simulink model "VSC_Grid_MyModel"  (R2017b)
settings: Solver=VariableStepAuto  StartTime=0.0  StopTime=5  MaxStep=1e-4  RelTol=1e-3  AbsTol=1e-3
PreLoadFcn:
  | VSC_Grid_Data_MyModel
values from neighbouring files (symbols this model uses):
  alpha_PQ = alpha_cc/10    (= 314.159265359)    [VSC_Grid_Data_MyModel.m]
  C_dc = 5000e-06    (= 0.005)    [VSC_Grid_Data_MyModel.m]
  D_low = 0.0001    [VSC_Grid_Data_MyModel.m]
  D_up = 0.9999    [VSC_Grid_Data_MyModel.m]
  fn = 50    [VSC_Grid_Data_MyModel.m]
  fnmax = 51    [VSC_Grid_Data_MyModel.m]
  fnmin = 49    [VSC_Grid_Data_MyModel.m]
  Kp_cc = alpha_cc*Lf    (= 6.28318530718)    [VSC_Grid_Data_MyModel.m]
  Kp_PLL = alpha_PLL*2    (= 62.8318530718)    [VSC_Grid_Data_MyModel.m]
  Lf = 2e-3    (= 0.002)    [VSC_Grid_Data_MyModel.m]
  R_dc = 1e-5    (= 1e-05)    [VSC_Grid_Data_MyModel.m]
  Rf = 6e-3    (= 0.006)    [VSC_Grid_Data_MyModel.m]
  samp_delay = 1.5*Ts    (= 0.0003)    [VSC_Grid_Data_MyModel.m]
  Ts = 2e-4    (= 0.0002)    [VSC_Grid_Data_MyModel.m]
  V_dc = 680    [VSC_Grid_Data_MyModel.m]
  VLL_rms = 230*sqrt(3)    [VSC_Grid_Data_MyModel.m]
undefined symbols (not defined in the file or in its folder): DiscIntNeverNeededParam, sigbuilder_block
libraries: powerlib x9, powerlib_meascontrol x4
settings Model: Creator=saioa  LastModifiedBy=saioa
settings DataIOCC: SaveFormat=Array  SaveOutput=off  SaveTime=off
settings OptimizationCC: LifeSpan=inf
settings DebuggingCC: UnconnectedInputMsg=none  UnconnectedOutputMsg=none  UnconnectedLineMsg=none

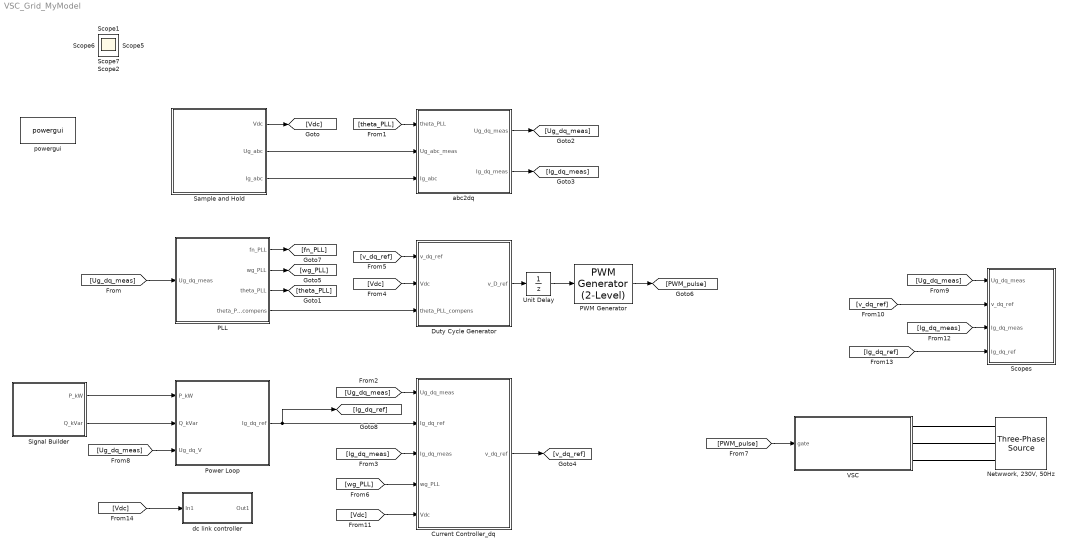
== system VSC_Grid_MyModel ==
  Current Controller_dq : Subsystem
  Duty Cycle Generator : Subsystem
  "Netwwork, 230V, 50Hz" : powerlib/Electrical Sources/Three-Phase Source  InternalConnection=Yg  VoltagePhases=off  Voltage=VLL_rms  PhaseAngle=0  Voltage_phases=[25e3 25e3 25e3]/sqrt(3)  PhaseAngles_phases=[0 -120 +120]  Frequency=fn  NonIdealSource=off  SpecifyImpedance=on  Resistance=0.8929  Inductance=16.58e-3  ShortCircuitLevel=40e6  BaseVoltage=600  XRratio=7  BusType=swing  Pref=0  Qref=0  Prefabc=[10e3, 10e3, 10e3]  Qrefabc=[0, 0, 0]  Qmin=-inf  Qmax=inf
  PLL : Subsystem
  PWM Generator : powerlib_meascontrol/Pulse & Signal Generators/PWM Generator (2-Level)  ModulatorType=Three-phase bridge (6 pulses)  ModulatorMode=Unsynchronized  Fc=fs  Pc=0  nF=27  MinMax="[ -1  1 ]"  SamplingTechnique=Symmetrical regular (single edge)  ModulatingSignals=off  m=0.8  Freq=60  Phase=0  Ts=0  ShowCarrierOutport=off
      settings: SourceProductName=Simscape Power Systems
  Power Loop : Subsystem
  Sample and Hold : Subsystem
  Scopes : Subsystem
  Signal Builder : Subsystem  Tag=STV Subsys  LoadFcn=sigbuilder_block('load');  StartFcn=sigbuilder_block('start');  StopFcn=sigbuilder_block('stop');  ClipboardFcn=sigbuilder_block('clipboard');  mask(Sigbuilder block){tuvar=[0:10]}
      mask help: Simulink:masks:SigbuilderBlock_MD
      mask init:
      | if ~strcmp(get_param(bdroot(gcbh),'SimulationStatus'),'stopped') tuvar = sigbuilder_block('maskInit'); end
      settings: CopyFcn=sigbuilder_block('copy');  DeleteFcn=sigbuilder_block('delete');  ModelCloseFcn=sigbuilder_block('modelClose');  PreSaveFcn=sigbuilder_block('preSave');  PauseFcn=sigbuilder_block('pause');  ContinueFcn=sigbuilder_block('continue');  NameChangeFcn=sigbuilder_block('namechange');  OpenFcn=sigbuilder_block('open',[6 33 1428 678 ]);  CloseFcn=sigbuilder_block('close');
      mask Display: plot(0, 0, 100, 100,[2, 2, 32, 32, 2], [68, 8, 8, 68, 68],[32, 2], [38, 38], [32, 19, 2],[53, 60, 44], [32, 17, 17, 2],[16, 16, 31, 31]);txt = getActiveGroup(gcbh);text(2, 100, txt,'verticalAlignment', 'top');
  Unit Delay : UnitDelay  SampleTime=-1
  VSC : Subsystem
  "abc2dq " : Subsystem
  dc link controller : Subsystem
  powergui : powerlib/powergui  Priority=1  SimulationMode=Continuous  SampleTime=50e-6  frequency=60  Iterations=50  frequencyindice=50  Pbase=100e6  ErrMax=1e-4  UnitsV=kV  UnitsW=MW  buscounter=0  FunctionMessages=off  echomessages=off  EnableUseOfTLC=off  CurrentSourceSwitches=off  DisableSnubberDevices=off  DisableRonSwitches=off  DisableVfSwitches=off  DisplayEquations=off  SolverType=Tustin/Backward Euler (TBE)  Interpol=off  ExternalGateDelay=off  methode=off  Ts=100  x0status=blocks  SPID=on  SwTol=0  HookPort=off  RestoreLinks=warning  ResistiveCurrentMeasurement=off  Frange=[0:2:500]  Ylog=off  Xlog=on  ShowGrid=off  save=off  variable=ZData  structure=0  ZoomFFT=off  StartTime=0.0  cycles=1  DisplayStyle=1  fundamental=60  FreqAxis=off  MaxFrequency=1000  frequencyindicesteady=1  RmsSteady=1  display=off
  Scope{,1..2,5..7} (6 alike) : Scope
  wires:
  "abc2dq "/2(Ig_dq_meas) -> [Ig_dq_meas]
  Sample and Hold/1(Vdc) -> [Vdc]
  Sample and Hold/3(Ig_abc) -> "abc2dq "/3(Ig_abc)
  [v_dq_ref] -> Duty Cycle Generator/1(v_dq_ref)
  PLL/4(theta_PLL_compens) -> Duty Cycle Generator/3(theta_PLL_compens)
  Current Controller_dq/1(v_dq_ref) -> [v_dq_ref]
  [Vdc] -> Duty Cycle Generator/2(Vdc)
  [Ug_dq_meas] -> Current Controller_dq/1(Ug_dq_meas)
  [theta_PLL] -> "abc2dq "/1(theta_PLL)
  "abc2dq "/1(Ug_dq_meas) -> [Ug_dq_meas]
  PLL/2(wg_PLL) -> [wg_PLL]
  [wg_PLL] -> Current Controller_dq/4(wg_PLL)
  PLL/1(fn_PLL) -> [fn_PLL]
  Sample and Hold/2(Ug_abc) -> "abc2dq "/2(Ug_abc_meas)
  PLL/3(theta_PLL) -> [theta_PLL]
  [Ug_dq_meas] -> PLL/1(Ug_dq_meas)
  [PWM_pulse] -> VSC/1(gate)
  Signal Builder/1(P_kW) -> Power Loop/1(P_kW)
  Signal Builder/2(Q_kVar) -> Power Loop/2(Q_kVar)
  [Ug_dq_meas] -> Power Loop/3(Ug_dq_V)
  Power Loop/1(Ig_dq_ref) -> Current Controller_dq/2(Ig_dq_ref), [Ig_dq_ref]
  [Ig_dq_meas] -> Current Controller_dq/3(Ig_dq_meas)
  [Vdc] -> Current Controller_dq/5(Vdc)
  PWM Generator/1 -> [PWM_pulse]
  Duty Cycle Generator/1(v_D_ref) -> Unit Delay/1
  Unit Delay/1 -> PWM Generator/1
  [Ug_dq_meas] -> Scopes/1(Ug_dq_meas)
  [v_dq_ref] -> Scopes/2(v_dq_ref)
  [Ig_dq_meas] -> Scopes/3(Ig_dq_meas)
  [Ig_dq_ref] -> Scopes/4(Ig_dq_ref)
  [Vdc] -> dc link controller/1(In1)
  connections:
  "Netwwork, 230V, 50Hz"/RConn1 -- VSC/RConn1
  "Netwwork, 230V, 50Hz"/RConn2 -- VSC/RConn2
  "Netwwork, 230V, 50Hz"/RConn3 -- VSC/RConn3

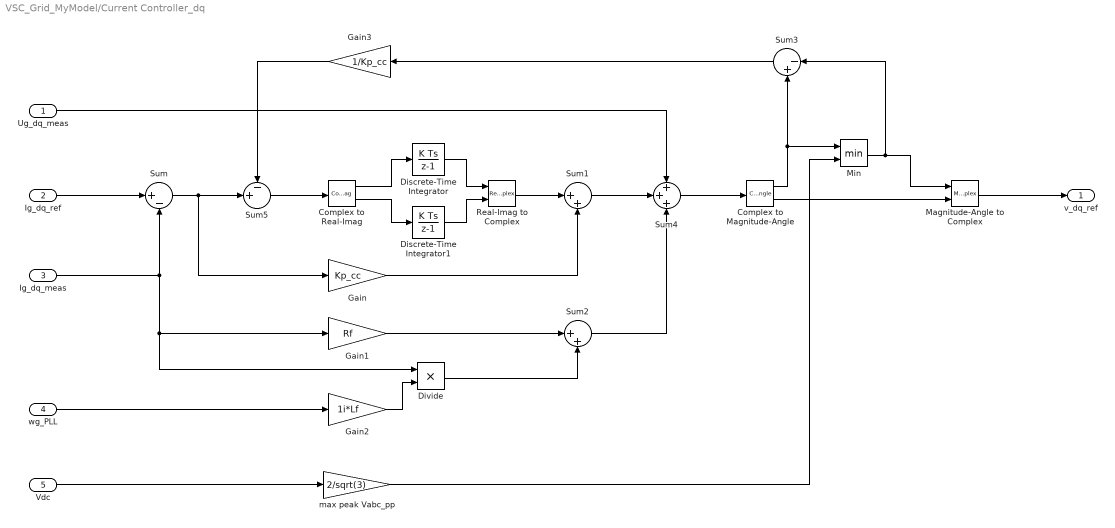
== system VSC_Grid_MyModel/Current Controller_dq ==
  Ug_dq_meas : Inport
  Ig_dq_ref : Inport  Port=2
  Ig_dq_meas : Inport  Port=3
  wg_PLL : Inport  Port=4
  Vdc : Inport  Port=5
  Complex to Magnitude-Angle : ComplexToMagnitudeAngle
  Complex to Real-Imag : ComplexToRealImag
  Discrete-Time Integrator : DiscreteIntegrator  gainval=Ki_cc  InitialConditionSetting=State (most efficient)  SampleTime=Ts  ICPrevOutput=DiscIntNeverNeededParam  ICPrevScaledInput=DiscIntNeverNeededParam
  Discrete-Time Integrator1 : DiscreteIntegrator  gainval=Ki_cc  InitialConditionSetting=State (most efficient)  SampleTime=Ts  ICPrevOutput=DiscIntNeverNeededParam  ICPrevScaledInput=DiscIntNeverNeededParam
  Divide : Product  Inputs=**
  Gain : Gain  Gain=Kp_cc
  Gain1 : Gain  Gain=Rf
  Gain2 : Gain  Gain=1i*Lf
  Gain3 : Gain  Gain=1/Kp_cc
  Magnitude-Angle to Complex : MagnitudeAngleToComplex
  Min : MinMax  Inputs=2
  Real-Imag to Complex : RealImagToComplex
  Sum : Sum  Inputs=|+-
  Sum1 : Sum  Inputs=|++
  Sum2 : Sum  Inputs=|++
  Sum3 : Sum  Inputs=|-+
  Sum4 : Sum  Inputs=+++  SaturateOnIntegerOverflow=on  InputSameDT=on  OutDataTypeStr=Inherit: Same as first input
  Sum5 : Sum  Inputs=-+|
  max peak Vabc_pp : Gain  Gain=2/sqrt(3)
  v_dq_ref : Outport
  wires:
  Ig_dq_meas/1 -> Gain1/1, Divide/1, Sum/2
  Ig_dq_ref/1 -> Sum/1
  Discrete-Time Integrator1/1 -> Real-Imag to Complex/2
  wg_PLL/1 -> Gain2/1
  Gain/1 -> Sum1/2
  Complex to Real-Imag/2 -> Discrete-Time Integrator1/1
  Discrete-Time Integrator/1 -> Real-Imag to Complex/1
  Real-Imag to Complex/1 -> Sum1/1
  Complex to Real-Imag/1 -> Discrete-Time Integrator/1
  Sum1/1 -> Sum4/2
  Sum2/1 -> Sum4/3
  Divide/1 -> Sum2/2
  Ug_dq_meas/1 -> Sum4/1
  Gain2/1 -> Divide/2
  Gain1/1 -> Sum2/1
  Vdc/1 -> max peak Vabc_pp/1
  Sum4/1 -> Complex to Magnitude-Angle/1
  Complex to Magnitude-Angle/1 -> Min/1, Sum3/2
  max peak Vabc_pp/1 -> Min/2
  Complex to Magnitude-Angle/2 -> Magnitude-Angle to Complex/2
  Min/1 -> Sum3/1, Magnitude-Angle to Complex/1
  Magnitude-Angle to Complex/1 -> v_dq_ref/1
  Sum5/1 -> Complex to Real-Imag/1
  Sum/1 -> Gain/1, Sum5/2
  Sum3/1 -> Gain3/1
  Gain3/1 -> Sum5/1

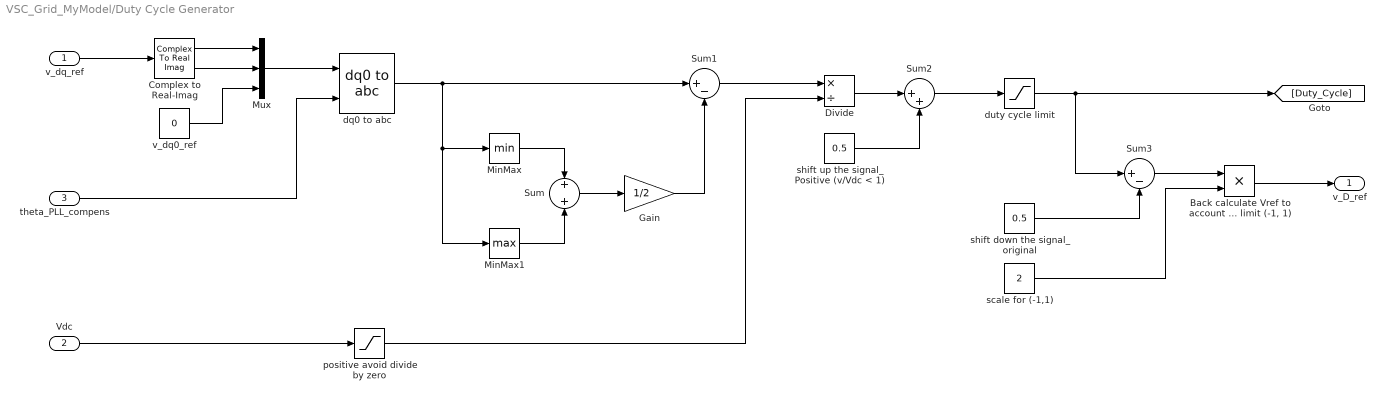
== system VSC_Grid_MyModel/Duty Cycle Generator ==
  v_dq_ref : Inport
  Vdc : Inport  Port=2
  theta_PLL_compens : Inport  Port=3
  "Back calculate Vref to account for duty cycle limit (-1, 1)" : Product  Inputs=**
  Complex to Real-Imag : ComplexToRealImag
  Divide : Product  Inputs=*/
  Gain : Gain  Gain=1/2
  MinMax : MinMax
  MinMax1 : MinMax  Function=max
  Mux : Mux  Inputs=3
  Sum : Sum  Inputs=+|+
  Sum1 : Sum  Inputs=|+-
  Sum2 : Sum  Inputs=|++
  Sum3 : Sum  Inputs=|+-
  dq0 to abc : powerlib_meascontrol/Transformations/dq0 to abc  Alignment=90 degrees behind phase A axis
  duty cycle limit : Saturate  UpperLimit=D_up  LowerLimit=D_low
  positive avoid divide by zero : Saturate  UpperLimit=inf  LowerLimit=1e-6
  scale for (-1,1) : Constant  Value=2
  shift down the signal_original : Constant  Value=0.5
  shift up the signal_Positive (v/Vdc < 1) : Constant  Value=0.5
  v_dq0_ref : Constant  Value=0
  v_D_ref : Outport
  wires:
  v_dq_ref/1 -> Complex to Real-Imag/1
  Complex to Real-Imag/1 -> Mux/1
  Complex to Real-Imag/2 -> Mux/2
  v_dq0_ref/1 -> Mux/3
  Mux/1 -> dq0 to abc/1
  theta_PLL_compens/1 -> dq0 to abc/2
  dq0 to abc/1 -> Sum1/1, MinMax1/1, MinMax/1
  Sum/1 -> Gain/1
  MinMax1/1 -> Sum/2
  MinMax/1 -> Sum/1
  Gain/1 -> Sum1/2
  Sum1/1 -> Divide/1
  Vdc/1 -> positive avoid divide by zero/1
  Divide/1 -> Sum2/1
  shift up the signal_Positive (v/Vdc < 1)/1 -> Sum2/2
  Sum2/1 -> duty cycle limit/1
  positive avoid divide by zero/1 -> Divide/2
  duty cycle limit/1 -> Sum3/1, [Duty_Cycle]
  shift down the signal_original/1 -> Sum3/2
  Sum3/1 -> "Back calculate Vref to account for duty cycle limit (-1, 1)"/1
  scale for (-1,1)/1 -> "Back calculate Vref to account for duty cycle limit (-1, 1)"/2
  "Back calculate Vref to account for duty cycle limit (-1, 1)"/1 -> v_D_ref/1

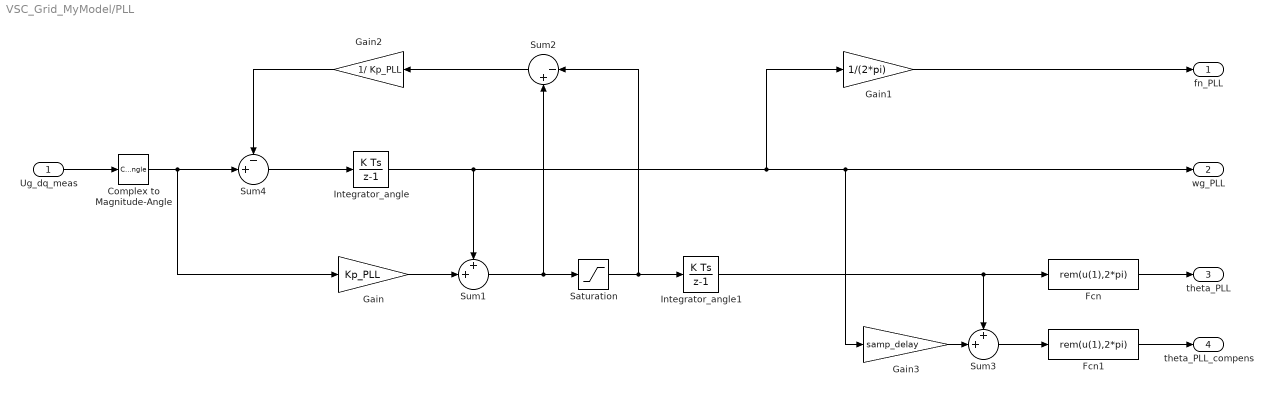
== system VSC_Grid_MyModel/PLL ==
  Ug_dq_meas : Inport
  Complex to Magnitude-Angle : ComplexToMagnitudeAngle  Output=Angle
  Fcn : Fcn  Expr=rem(u(1),2*pi)
  Fcn1 : Fcn  Expr=rem(u(1),2*pi)
  Gain : Gain  Gain=Kp_PLL
  Gain1 : Gain  Gain=1/(2*pi)
  Gain2 : Gain  Gain=1/ Kp_PLL
  Gain3 : Gain  Gain=samp_delay
  Integrator_angle : DiscreteIntegrator  gainval=Ki_PLL  InitialCondition=2*pi*fn  InitialConditionSetting=State (most efficient)  SampleTime=Ts  ICPrevOutput=DiscIntNeverNeededParam  ICPrevScaledInput=DiscIntNeverNeededParam
  Integrator_angle1 : DiscreteIntegrator  gainval=1  InitialConditionSetting=State (most efficient)  SampleTime=Ts  ICPrevOutput=DiscIntNeverNeededParam  ICPrevScaledInput=DiscIntNeverNeededParam
  Saturation : Saturate  UpperLimit=2*pi*fnmax  LowerLimit=2*pi*fnmin
  Sum1 : Sum  Inputs=++|
  Sum2 : Sum  Inputs=|-+
  Sum3 : Sum  Inputs=++|
  Sum4 : Sum  Inputs=-+|
  fn_PLL : Outport
  wg_PLL : Outport  Port=2
  theta_PLL : Outport  Port=3
  theta_PLL_compens : Outport  Port=4
  wires:
  Ug_dq_meas/1 -> Complex to Magnitude-Angle/1
  Integrator_angle/1 -> Gain1/1, wg_PLL/1, Gain3/1, Sum1/1
  Complex to Magnitude-Angle/1 -> Sum4/2, Gain/1
  Sum1/1 -> Sum2/2, Saturation/1
  Gain/1 -> Sum1/2
  Integrator_angle1/1 -> Sum3/1, Fcn/1
  Gain1/1 -> fn_PLL/1
  Fcn/1 -> theta_PLL/1
  Sum3/1 -> Fcn1/1
  Gain3/1 -> Sum3/2
  Fcn1/1 -> theta_PLL_compens/1
  Saturation/1 -> Sum2/1, Integrator_angle1/1
  Sum2/1 -> Gain2/1
  Sum4/1 -> Integrator_angle/1
  Gain2/1 -> Sum4/1

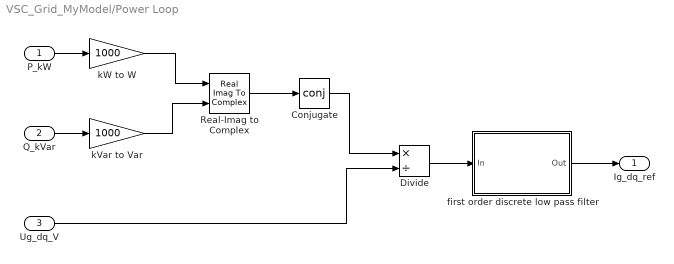
== system VSC_Grid_MyModel/Power Loop ==
  P_kW : Inport
  Q_kVar : Inport  Port=2
  Ug_dq_V : Inport  Port=3
  Conjugate : Math  Operator=conj  RndMeth=Zero  SaturateOnIntegerOverflow=on
  Divide : Product  Inputs=*/
  Real-Imag to Complex : RealImagToComplex
  first order discrete low pass filter : Subsystem  mask(First-order low pass filter (Discrete)){alpha_wfilter=alpha_PQ, Ts=Ts, Init=0}
      mask prompts: alpha_wfilter "Bandwidth (rad/s)"; Ts "Sampling time (>0, s)"; Init "Initial condition"
      mask help: Forward Euler method
  kVar to Var : Gain  Gain=1000
  kW to W : Gain  Gain=1000
  Ig_dq_ref : Outport
  wires:
  Divide/1 -> first order discrete low pass filter/1(In)
  Real-Imag to Complex/1 -> Conjugate/1
  Q_kVar/1 -> kVar to Var/1
  P_kW/1 -> kW to W/1
  Ug_dq_V/1 -> Divide/2
  Conjugate/1 -> Divide/1
  kW to W/1 -> Real-Imag to Complex/1
  kVar to Var/1 -> Real-Imag to Complex/2
  first order discrete low pass filter/1(Out) -> Ig_dq_ref/1

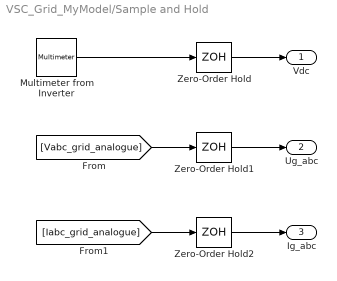
== system VSC_Grid_MyModel/Sample and Hold ==
  "Multimeter from Inverter " : powerlib/Measurements/Multimeter  PhasorSimulation=off  OutputType=Complex  sel=10  L=16  Gain=1  yselected="{'Udc: VSC/PWM  IGBT Inverter'};"  PSBOutputType=1  PSBequivalent=0  AxesSetting=[0,0.1,-100,100]  Display=0  SavedBlockNames=-11
  Zero-Order Hold : ZeroOrderHold  SampleTime=Ts
  Zero-Order Hold1 : ZeroOrderHold  SampleTime=Ts
  Zero-Order Hold2 : ZeroOrderHold  SampleTime=Ts
  Vdc : Outport
  Ug_abc : Outport  Port=2
  Ig_abc : Outport  Port=3
  wires:
  Zero-Order Hold/1 -> Vdc/1
  "Multimeter from Inverter "/1 -> Zero-Order Hold/1
  [Vabc_grid_analogue] -> Zero-Order Hold1/1
  [Iabc_grid_analogue] -> Zero-Order Hold2/1
  Zero-Order Hold1/1 -> Ug_abc/1
  Zero-Order Hold2/1 -> Ig_abc/1

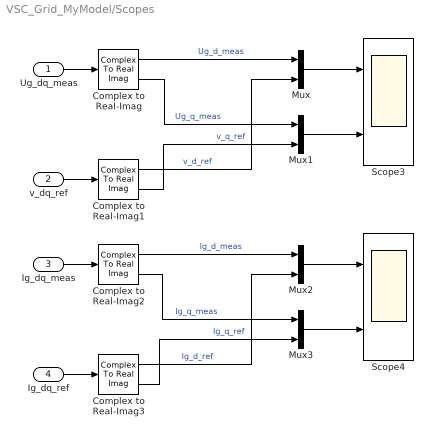
== system VSC_Grid_MyModel/Scopes ==
  Ug_dq_meas : Inport
  v_dq_ref : Inport  Port=2
  Ig_dq_meas : Inport  Port=3
  Ig_dq_ref : Inport  Port=4
  Complex to Real-Imag{,1..3} (4 alike) : ComplexToRealImag
  Mux{,1..3} (4 alike) : Mux  Inputs=2
  Scope3 : Scope  NumInputPorts=2
  Scope4 : Scope  NumInputPorts=2
  wires:
  Complex to Real-Imag3/2 -> Mux3/2  "Ig_q_ref"
  Ig_dq_ref/1 -> Complex to Real-Imag3/1
  Mux3/1 -> Scope4/2
  Complex to Real-Imag2/1 -> Mux2/1  "Ig_d_meas"
  Mux2/1 -> Scope4/1
  Mux1/1 -> Scope3/2
  Ig_dq_meas/1 -> Complex to Real-Imag2/1
  Complex to Real-Imag/2 -> Mux1/1  "Ug_q_meas"
  Complex to Real-Imag3/1 -> Mux2/2  "Ig_d_ref"
  Complex to Real-Imag1/2 -> Mux1/2  "v_q_ref"
  Complex to Real-Imag/1 -> Mux/1  "Ug_d_meas"
  Complex to Real-Imag2/2 -> Mux3/1  "Ig_q_meas"
  v_dq_ref/1 -> Complex to Real-Imag1/1
  Mux/1 -> Scope3/1
  Complex to Real-Imag1/1 -> Mux/2  "v_d_ref"
  Ug_dq_meas/1 -> Complex to Real-Imag/1

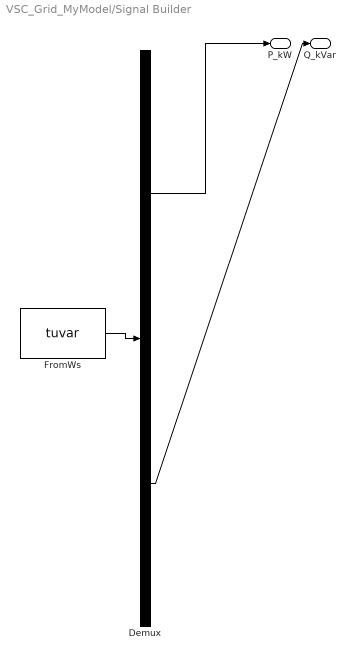
== system VSC_Grid_MyModel/Signal Builder ==
  Demux : Demux  Tag=STV Demux  Outputs=2
  FromWs : FromWorkspace  Tag=STV FromWs  VariableName=tuvar  SampleTime=0
      SigBuilderData=|
      | common.afterFinalStr = 'Extrapolate'
      | common.sampleTime = 0
      | dataSet(1).timeRange = [0 10]
      | dataSet(1).name = 'Zero_Power'
      | dataSet(2).timeRange = [0 10]
      | dataSet(2).name = 'Power Step'
      | sbobj.Groups(1).Name = 'Zero_Power'
      | sbobj.Groups(1).Signals(1).Name = 'P_kW'
      | sbobj.Groups(1).Signals(1).XData = [0 10]
      | sbobj.Groups(1).Signals(1).YData = [0 0]
      | sbobj.Groups(1).Signals(2).Name = 'Q_kVar'
      | sbobj.Groups(1).Signals(2).XData = [0 10]
      | sbobj.Groups(1).Signals(2).YData = [0 0]
      | sbobj.Groups(2).Name = 'Power Step'
      | sbobj.Groups(2).Signals(1).Name = 'P_kW'
      | sbobj.Groups(2).Signals(1).XData = [0 2.5 2.5 10]
      | sbobj.Groups(2).Signals(1).YData = [0 0 35 35]
      | sbobj.Groups(2).Signals(2).Name = 'Q_kVar'
      | sbobj.Groups(2).Signals(2).XData = [0 10]
      | sbobj.Groups(2).Signals(2).YData = [0 0]
  P_kW : Outport  Tag=STV Outport
  Q_kVar : Outport  Tag=STV Outport  Port=2
  wires:
  Demux/1 -> P_kW/1
  FromWs/1 -> Demux/1
  Demux/2 -> Q_kVar/1

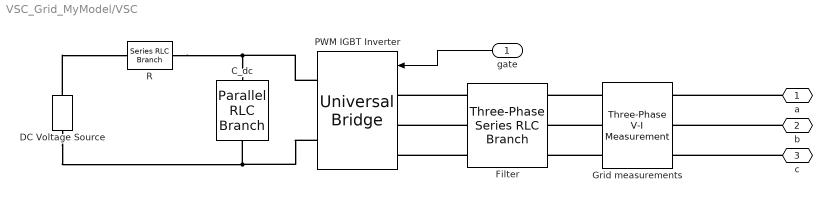
== system VSC_Grid_MyModel/VSC ==
  gate : Inport
  C_dc : powerlib/Elements/Parallel RLC Branch  LConnTagsString=a  RConnTagsString=__new0  BranchType=C  Resistance=1  Inductance=1e-3  SetiL0=off  InitialCurrent=0  Capacitance=C_dc  Setx0=off  InitialVoltage=0  Measurements=None
  DC Voltage Source : powerlib/Electrical Sources/DC Voltage Source  Amplitude=V_dc  Measurements=None
  Filter : powerlib/Elements/Three-Phase Series RLC Branch  LConnTagsString=A|B|C  RConnTagsString=A|B|C  BranchType=RL  Resistance=Rf  Inductance=Lf  Capacitance=1e-6  Measurements=None
  Grid measurements : powerlib/Measurements/Three-Phase V-I Measurement  VoltageMeasurement=phase-to-ground  SetLabelV=on  LabelV=Vabc_grid_analogue  Vpu=off  VpuLL=off  CurrentMeasurement=yes  SetLabelI=on  LabelI=Iabc_grid_analogue  Ipu=off  Pbase=100e6  Vbase=500e3  OutputType=Complex  PhasorSimulation=off  PSBequivalent=0
  PWM IGBT Inverter : powerlib/Power Electronics/Universal Bridge  Arms=3  SnubberResistance=Rs  SnubberCapacitance=Cs  Device=IGBT / Diodes  Ron=Ron  Lon=0  ForwardVoltages="[  0.0  0.0  ]"  ForwardVoltage=.8  GTOparameters=[ 1e-6 ,1e-6 ]  IGBTparameters=[ 1e-6 , 2e-6 ]  Measurements=All voltages and currents  Measurements_2=None  converterType=Rectifier
  R : powerlib/Elements/Series RLC Branch  LConnTagsString=__new0  RConnTagsString=__new0  BranchType=R  Resistance=R_dc  Inductance=1e-3  SetiL0=off  InitialCurrent=0  Capacitance=1e-6  Setx0=off  InitialVoltage=0  Measurements=None
  a : PMIOPort  Port=1  Side=Right
  b : PMIOPort  Port=2  Side=Right
  c : PMIOPort  Port=3  Side=Right
  wires:
  gate/1 -> PWM IGBT Inverter/1
  connections:
  DC Voltage Source/RConn1 -- R/LConn1
  DC Voltage Source/LConn1 -- PWM IGBT Inverter/RConn2 -- C_dc/RConn1
  Filter/LConn2 -- PWM IGBT Inverter/LConn2
  Filter/LConn3 -- PWM IGBT Inverter/LConn3
  Filter/LConn1 -- PWM IGBT Inverter/LConn1
  R/RConn1 -- C_dc/LConn1 -- PWM IGBT Inverter/RConn1
  b/RConn1 -- Grid measurements/RConn2
  Grid measurements/LConn2 -- Filter/RConn2
  Grid measurements/LConn1 -- Filter/RConn1
  Grid measurements/LConn3 -- Filter/RConn3
  c/RConn1 -- Grid measurements/RConn3
  a/RConn1 -- Grid measurements/RConn1

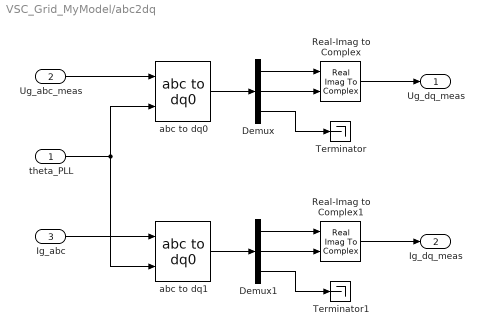
== system VSC_Grid_MyModel/abc2dq  ==
  theta_PLL : Inport
  Ug_abc_meas : Inport  Port=2
  Ig_abc : Inport  Port=3
  Demux : Demux  Outputs=3
  Demux1 : Demux  Outputs=3
  Real-Imag to Complex : RealImagToComplex
  Real-Imag to Complex1 : RealImagToComplex
  Terminator : Terminator
  Terminator1 : Terminator
  abc to dq0 : powerlib_meascontrol/Transformations/abc to dq0  Alignment=90 degrees behind phase A axis
  abc to dq1 : powerlib_meascontrol/Transformations/abc to dq0  Alignment=90 degrees behind phase A axis
  Ug_dq_meas : Outport
  Ig_dq_meas : Outport  Port=2
  wires:
  Ug_abc_meas/1 -> abc to dq0/1
  theta_PLL/1 -> abc to dq1/2, abc to dq0/2
  Ig_abc/1 -> abc to dq1/1
  abc to dq0/1 -> Demux/1
  Demux/2 -> Real-Imag to Complex/2
  Demux/1 -> Real-Imag to Complex/1
  Real-Imag to Complex/1 -> Ug_dq_meas/1
  Demux/3 -> Terminator/1
  abc to dq1/1 -> Demux1/1
  Demux1/2 -> Real-Imag to Complex1/2
  Demux1/3 -> Terminator1/1
  Real-Imag to Complex1/1 -> Ig_dq_meas/1
  Demux1/1 -> Real-Imag to Complex1/1

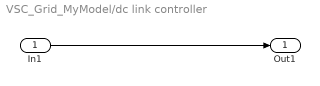
== system VSC_Grid_MyModel/dc link controller ==
  In1 : Inport
  Out1 : Outport
  wires:
  In1/1 -> Out1/1

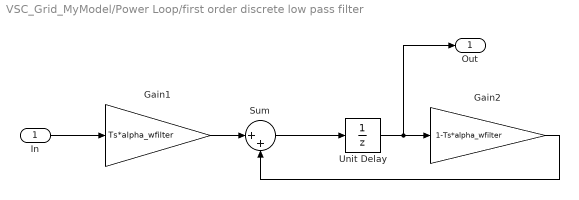
== system VSC_Grid_MyModel/Power Loop/first order discrete low pass filter ==
  In : Inport
  Gain1 : Gain  Gain=Ts*alpha_wfilter
  Gain2 : Gain  Gain=1-Ts*alpha_wfilter
  Sum : Sum  Inputs=|++
  Unit Delay : UnitDelay  InitialCondition=Init  SampleTime=Ts
  Out : Outport
  wires:
  Gain2/1 -> Sum/2
  In/1 -> Gain1/1
  Sum/1 -> Unit Delay/1
  Gain1/1 -> Sum/1
  Unit Delay/1 -> Out/1, Gain2/1
